simulink model "CM"  (R2020a)
settings: Solver=ode45  StartTime=0.0  StopTime=100  RelTol=1e-3  EnableMultiTasking=on
undefined symbols (not defined in the file or in its folder): DiscIntNeverNeededParam
libraries: simulink x3, rllib x1
settings Model: Creator=The MathWorks, Inc.  LastModifiedBy=badit
settings DataIOCC: LimitDataPoints=on  SaveFormat=Array  SignalLoggingName=logsOut
settings OptimizationCC: ExpressionDepthLimit=2147483647  InitFltsAndDblsToZero=on  LifeSpan=inf
settings DebuggingCC: SaveWithParameterizedLinksMsg=none  UnderspecifiedInitializationDetection=Classic  MergeDetectMultiDrivingBlocksExec=none  SignalResolutionControl=TryResolveAllWithWarning  MultiTaskDSMMsg=warning  FcnCallInpInsideContextMsg=warning  AllowSymbolicDim=off  StateNameClashWarn=warning  SFUnexpectedBacktrackingDiag=warning  SFNoUnconditionalDefaultTransitionDiag=warning  SFExecutionAtInitializationDiag=none  ArithmeticOperatorsInVariantConditions=warning
settings HardwareCC: ProdBitPerPointer=32  ProdBitPerSizeT=32  ProdBitPerPtrDiffT=32  ProdLargestAtomicFloat=None  ProdIntDivRoundTo=Undefined  ProdEndianess=Unspecified  ProdWordSize=32  ProdHWDeviceType=Specified
settings ModelReferenceCC: PropagateSignalLabelsOutOfModel=off
settings SFSimCC: SimUseLocalCustomCode=off  CustomCodeUndefinedFunction=UseInterfaceOnly
settings RTWCC: RTWUseLocalCustomCode=off
settings CodeAppCC: StateflowObjectComments=on
settings GRTTargetCC: TargetFcnLib=ansi_tfl_tmw.mat  TargetLangStandard=C89/C90 (ANSI)  CombineOutputUpdateFcns=off  GRTInterface=on
settings ConfigComp: CovMetricSettings=dw  CovHtmlReporting=on  CovSaveCumulativeToWorkspaceVar=on  CovSaveSingleToWorkspaceVar=on  CovExternalEMLEnable=off

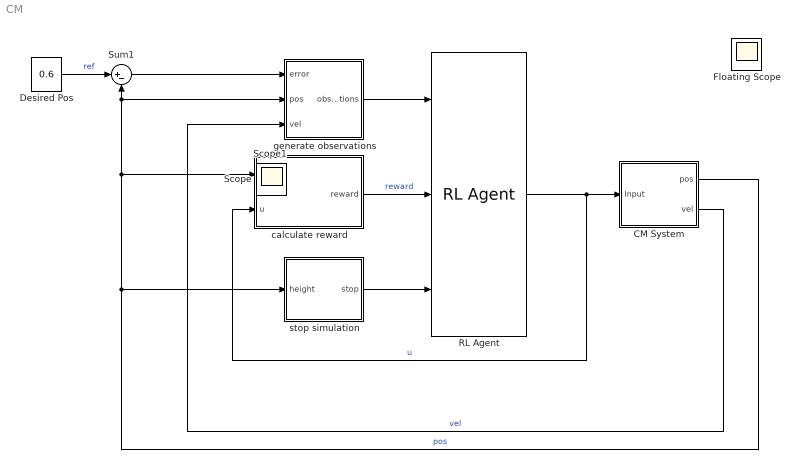
== system CM ==
  CM System : Subsystem
  Desired Pos : Constant  Value=0.6
  Floating Scope : Scope
      settings: Floating=on
  RL Agent : rllib/RL Agent  Agent=agent  ProvideReward=on  ProvideIsDone=on  ProvideCumRwd=off  TreatAsDirectFeedthrough=on  CollectLoggedSignals=on  CollectModelStates=on
  Sum1 : Sum  Inputs=|+-  SaturateOnIntegerOverflow=on
  calculate reward : Subsystem
  generate observations : Subsystem
  stop simulation : Subsystem
  Scope : Scope
  Scope1 : Scope
  wires:
  Desired Pos/1 -> Sum1/1  "ref"
  CM System/1(pos) -> generate observations/2(pos), Sum1/2, calculate reward/1(pos), stop simulation/1(height)  "pos"
  RL Agent/1 -> calculate reward/2(u), CM System/1(Input)  "u"
  stop simulation/1(stop) -> RL Agent/3
  calculate reward/1(reward) -> RL Agent/2  "reward"
  generate observations/1(observations) -> RL Agent/1
  CM System/2(vel) -> generate observations/3(vel)  "vel"
  Sum1/1 -> generate observations/1(error)

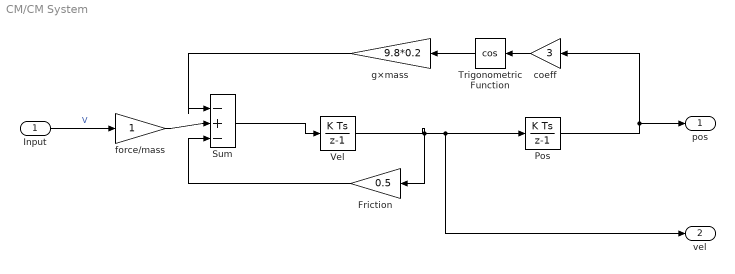
== system CM/CM System ==
  Input : Inport
  Friction : Gain  Gain=0.5  SaturateOnIntegerOverflow=on  OutDataTypeStr=Inherit: Same as input  ParamDataTypeStr=Inherit: Same as input
  Pos : DiscreteIntegrator  InitialCondition=0.6  SampleTime=-1  LimitOutput=on  UpperSaturationLimit=0.6  LowerSaturationLimit=-1.2  ICPrevOutput=DiscIntNeverNeededParam  ICPrevScaledInput=DiscIntNeverNeededParam
  Sum : Sum  Inputs=|-+-  SaturateOnIntegerOverflow=on
  Trigonometric Function : Trigonometry  Operator=cos
  Vel : DiscreteIntegrator  InitialCondition=0.42  SampleTime=-1  LimitOutput=on  UpperSaturationLimit=1.5  LowerSaturationLimit=-1.5  ICPrevOutput=DiscIntNeverNeededParam  ICPrevScaledInput=DiscIntNeverNeededParam
  coeff : Gain  Gain=3  SaturateOnIntegerOverflow=on  OutDataTypeStr=Inherit: Same as input  ParamDataTypeStr=Inherit: Same as input
  force/mass : Gain  SaturateOnIntegerOverflow=on  OutDataTypeStr=Inherit: Same as input  ParamDataTypeStr=Inherit: Same as input
  g×mass : Gain  Gain=9.8*0.2  SaturateOnIntegerOverflow=on  OutDataTypeStr=Inherit: Same as input  ParamDataTypeStr=Inherit: Same as input
  pos : Outport  VectorParamsAs1DForOutWhenUnconnected=off
  vel : Outport  Port=2  VectorParamsAs1DForOutWhenUnconnected=off
  wires:
  Input/1 -> force/mass/1  "V"
  Pos/1 -> pos/1, coeff/1
  Trigonometric Function/1 -> g×mass/1
  Friction/1 -> Sum/3
  force/mass/1 -> Sum/2
  Sum/1 -> Vel/1
  g×mass/1 -> Sum/1
  coeff/1 -> Trigonometric Function/1
  Vel/1 -> vel/1, Pos/1, Friction/1

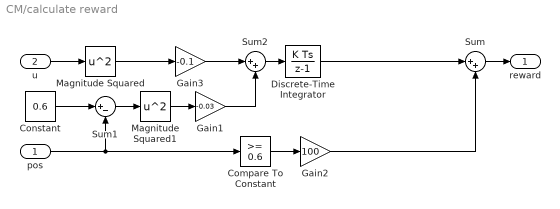
== system CM/calculate reward ==
  pos : Inport
  u : Inport  Port=2
  Compare To Constant : simulink/Logic and Bit Operations/Compare To Constant  relop=>=  const=0.6  OutDataTypeStr=boolean
  Constant : Constant  Value=0.6
  Discrete-Time Integrator : DiscreteIntegrator  SampleTime=-1  ICPrevOutput=DiscIntNeverNeededParam  ICPrevScaledInput=DiscIntNeverNeededParam
  Gain1 : Gain  Gain=-0.03
  Gain2 : Gain  Gain=100
  Gain3 : Gain  Gain=-0.1
  Magnitude Squared : Math  Operator=square  SignedPower=on  OutputSignalType=real  SaturateOnIntegerOverflow=on
  Magnitude Squared1 : Math  Operator=square  SignedPower=on  OutputSignalType=real  SaturateOnIntegerOverflow=on
  Sum : Sum  Inputs=|++  OutDataTypeStr=double
  Sum1 : Sum  Inputs=|+-  OutDataTypeStr=double
  Sum2 : Sum  Inputs=|++  OutDataTypeStr=double
  reward : Outport  VectorParamsAs1DForOutWhenUnconnected=off
  wires:
  pos/1 -> Sum1/2, Compare To Constant/1
  Sum/1 -> reward/1
  Compare To Constant/1 -> Gain2/1
  Gain2/1 -> Sum/2
  Sum2/1 -> Discrete-Time Integrator/1
  u/1 -> Magnitude Squared/1
  Constant/1 -> Sum1/1
  Sum1/1 -> Magnitude Squared1/1
  Magnitude Squared1/1 -> Gain1/1
  Magnitude Squared/1 -> Gain3/1
  Gain3/1 -> Sum2/1
  Gain1/1 -> Sum2/2
  Discrete-Time Integrator/1 -> Sum/1

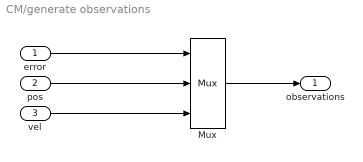
== system CM/generate observations ==
  error : Inport
  pos : Inport  Port=2
  vel : Inport  Port=3
  Mux : Mux  Inputs=3
  observations : Outport  VectorParamsAs1DForOutWhenUnconnected=off
  wires:
  Mux/1 -> observations/1
  pos/1 -> Mux/2
  vel/1 -> Mux/3
  error/1 -> Mux/1

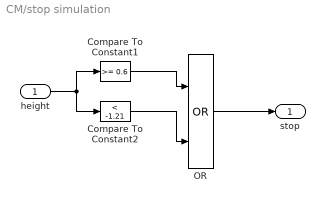
== system CM/stop simulation ==
  height : Inport
  Compare To Constant1 : simulink/Logic and Bit Operations/Compare To Constant  relop=>=  const=0.6  OutDataTypeStr=boolean
  Compare To Constant2 : simulink/Logic and Bit Operations/Compare To Constant  relop=<  const=-1.21  OutDataTypeStr=boolean
  OR : Logic  Operator=OR  IconShape=distinctive  AllPortsSameDT=off  OutDataTypeStr=boolean
  stop : Outport  VectorParamsAs1DForOutWhenUnconnected=off
  wires:
  height/1 -> Compare To Constant2/1, Compare To Constant1/1
  Compare To Constant2/1 -> OR/2
  Compare To Constant1/1 -> OR/1
  OR/1 -> stop/1
